simulink model "Planner_Operational_Space"  (Simulink 9.2)
settings: Solver=FixedStepDiscrete  StartTime=0.0  StopTime=stop_time  FixedStep=dt  RelTol=1e-3  EnableMultiTasking=on
values from neighbouring files (symbols this model uses):
  c1 = ((a1+a2*c2)*pw_x+a2*s2*pw_y)/(pw_x^2+pw_y^2)    [analitycal_IK_4DoF_v1.m]    (also in initialization_simulazione.m = [25 49.5]; provatraiettoria.m = [25 49.5])
  c2 = (pw_x^2+pw_y^2-a1^2-a2^2)/(2*a1*a2)    [analitycal_IK_4DoF_v1.m]    (also in initialization_simulazione.m = [25 11]; provatraiettoria.m = [25 11])
  r1 = 30    [initialization_simulazione.m]    (also in provatraiettoria.m)
  r2 = 10    [initialization_simulazione.m]    (also in provatraiettoria.m)
undefined symbols (not defined in the file or in its folder): planner_TOAD
libraries: simulink x1
settings Model: Creator=Nino  LastModifiedBy=cecil
settings OptimizationCC: ExpressionDepthLimit=2147483647  InitFltsAndDblsToZero=on
settings DebuggingCC: SolverPrmCheckMsg=warning
settings ConfigComp: CovSFcnEnable=off

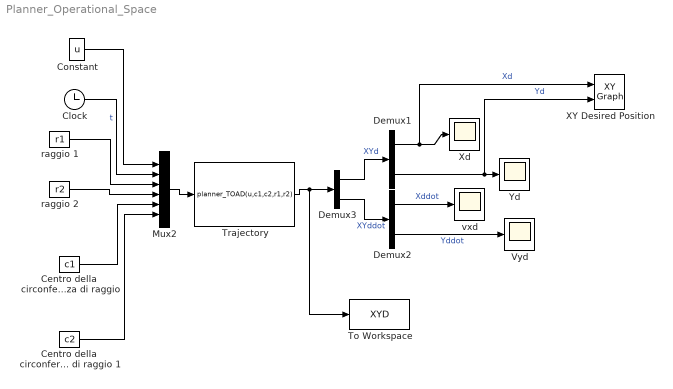
== system Planner_Operational_Space ==
  "Centro della  circonferenza di raggio " : Constant  Value=c1
  Centro della  circonferenza di raggio 1 : Constant  Value=c2
  Clock : Clock
  Constant : Constant  Value=u
  Demux1 : Demux  Outputs=2
  Demux2 : Demux  Outputs=2
  Demux3 : Demux  Outputs=2
  Mux2 : Mux  Inputs=6
  To Workspace : ToWorkspace  VariableName=XYD  SaveFormat=Structure  SampleTime=-1
  Trajectory : MATLABFcn  MATLABFcn=planner_TOAD(u,c1,c2,r1,r2)  OutputDimensions=4
  Vyd : Scope
  XY Desired Position : simulink/Sinks/XY Graph  xmin=-0.2  xmax=0.2  ymin=-0.2  ymax=0.2  st=-1
  Xd : Scope
  Yd : Scope
  raggio 1 : Constant  Value=r1
  raggio 2 : Constant  Value=r2
  vxd : Scope
  wires:
  Demux2/2 -> Vyd/1  "Yddot"
  Demux2/1 -> vxd/1  "Xddot"
  Demux1/2 -> Yd/1, XY Desired Position/2  "Yd"
  Demux1/1 -> Xd/1, XY Desired Position/1  "Xd"
  Demux3/1 -> Demux1/1  "XYd"
  Demux3/2 -> Demux2/1  "XYddot"
  Trajectory/1 -> Demux3/1, To Workspace/1
  Mux2/1 -> Trajectory/1
  Constant/1 -> Mux2/1
  Clock/1 -> Mux2/2  "t"
  "Centro della  circonferenza di raggio "/1 -> Mux2/5
  Centro della  circonferenza di raggio 1/1 -> Mux2/6
  raggio 1/1 -> Mux2/3
  raggio 2/1 -> Mux2/4
